simulink model "TxSteering_RxMVDR_4x4_HDL_IQ"  (R2020a)
settings: Solver=FixedStepDiscrete  StartTime=0.0  StopTime=stoptime*0 + inf  RelTol=1e-3
PreLoadFcn:
  | load('iq_bus_obj.mat');
  | model_init
InitFcn:
  | model_init
model workspace (MAT data in the model file):
  socvcb : containers.Map (value not decoded)
values from neighbouring files (symbols this model uses):
  BackSubstitutePrototype = fi(0, matrixdivbacksub_dt)    [model_init.m]
  DataSampleRate = ConverterSampleRate/DecimInterpFactor    (= 245760000)    [model_init.m]
  fc = ConverterSampleRate/4    (= 491520000)    [model_init.m]
  FPGAClkRate = DataSampleRate/VectorSamplingFactor    (= 245760000)    [model_init.m]
  matrixDivDelay = NumberOfCORDICIterations*10 + 86    [model_init.m]
  movavg_bitshift = nextpow2(sqrt(windowSize))    [model_init.m]
  mvdrPipelineDelay = covMatDelay+movAvgDelay+matrixDivDelay+normResponseDelay    [model_init.m]
  NCO_bits = 14    [model_init.m]
  numArrayElements = 4    [model_init.m]
  NumberOfCORDICIterations = matrixdivin_dt.WordLength - 1    [model_init.m]
  S2MM_frame_size = FrameSize*4    (= 40000)    [host_io_init.m]    (also in model_init.m = 1000)
  windowSize = 1024    [model_init.m]
undefined symbols (not defined in the file or in its folder): Fo, Fs, N, physconst
libraries: hdlsllib x268, simulink x53, dspsolvers x1, embreciprocals x1, dsphdlsigops x1
(part 2 of 12)

== system TxSteering_RxMVDR_4x4_HDL_IQ/DUT/Tx Signal Generation/ConcatADCChannels ==
  "Tile1_Ch1_I_Data " : Inport
  Tile1_Ch1_Q_Data : Inport  Port=2
  Tile1_Ch2_I_Data : Inport  Port=3
  Tile1_Ch2_Q_Data : Inport  Port=4
  Tile2_Ch1_I_Data : Inport  Port=5
  Tile2_Ch1_Q_Data : Inport  Port=6
  Tile2_Ch2_I_Data : Inport  Port=7
  Tile2_Ch2_Q_Data : Inport  Port=8
  Valid : Inport  Port=9
  Data Type Conversion : DataTypeConversion  OutDataTypeStr=input_dt  ConvertRealWorld=Stored Integer (SI)
  Real-Imag to Complex{,1..3} (4 alike) : RealImagToComplex
  To Data Bus : Subsystem  mask(To Data Bus){dummy=0}
      mask help: Create a streaming Data Bus from Data and Valid signals.
      mask Display:
      | port_label('input',1,'data');
      | port_label('input',2,'valid');
  Vector Concatenate : Concatenate  NumInputs=4  Mode=Multidimensional array  ConcatenateDimension=2
  DataBusOut : Outport  VectorParamsAs1DForOutWhenUnconnected=off
  wires:
  Real-Imag to Complex/1 -> Vector Concatenate/1
  Real-Imag to Complex1/1 -> Vector Concatenate/2
  Real-Imag to Complex2/1 -> Vector Concatenate/3
  Real-Imag to Complex3/1 -> Vector Concatenate/4
  Vector Concatenate/1 -> Data Type Conversion/1
  Valid/1 -> To Data Bus/2(valid)
  Data Type Conversion/1 -> To Data Bus/1(data)
  To Data Bus/1(bus) -> DataBusOut/1
  "Tile1_Ch1_I_Data "/1 -> Real-Imag to Complex/1
  Tile1_Ch1_Q_Data/1 -> Real-Imag to Complex/2
  Tile1_Ch2_I_Data/1 -> Real-Imag to Complex1/1
  Tile1_Ch2_Q_Data/1 -> Real-Imag to Complex1/2
  Tile2_Ch1_I_Data/1 -> Real-Imag to Complex2/1
  Tile2_Ch1_Q_Data/1 -> Real-Imag to Complex2/2
  Tile2_Ch2_I_Data/1 -> Real-Imag to Complex3/1
  Tile2_Ch2_Q_Data/1 -> Real-Imag to Complex3/2

== system TxSteering_RxMVDR_4x4_HDL_IQ/DUT/Tx Signal Generation/Generate Steering Channels ==
  increment : Inport  Partition=on  PartitionDimension=1  PartitionWidth=1  PartitionOffset=0
  gain : Inport  Port=2  Partition=on  PartitionDimension=1  PartitionWidth=1  PartitionOffset=0
  steeringCoeffs : Inport  Port=3  Partition=on  PartitionDimension=1  PartitionWidth=4  PartitionOffset=0
  Apply Steering Coefficients : Subsystem  TreatAsAtomicUnit=on
  Data Type Conversion : DataTypeConversion  OutDataTypeStr=fixdt(1,16,0)
  For Each : ForEach  DisableCoverage=on
  NCO : Subsystem
  Selector : Selector  InputPortWidth=4  IndexOptions=Index vector (dialog)  Indices=1  OutputSizes=1
  dataOut : Outport  ConcatenationDimension=1
  validOut : Outport  Port=2  ConcatenationDimension=1
  wires:
  Data Type Conversion/1 -> dataOut/1
  Selector/1 -> validOut/1
  steeringCoeffs/1 -> Apply Steering Coefficients/3(coeffIn)
  increment/1 -> NCO/1(increment)
  Apply Steering Coefficients/1(dataOut) -> Data Type Conversion/1
  Apply Steering Coefficients/2(validOut) -> Selector/1
  NCO/1(dataOut) -> Apply Steering Coefficients/1(dataIn)
  gain/1 -> NCO/2(gain)
  NCO/2(validOut) -> Apply Steering Coefficients/2(validIn)

== system TxSteering_RxMVDR_4x4_HDL_IQ/AXI4Stream_DMA_S2MM/ForCalibration/Unpack Complex/For Each Subsystem ==
  In1 : Inport  Partition=on  PartitionDimension=1  PartitionWidth=1  PartitionOffset=0
  For Each : ForEach  DisableCoverage=on
  Out1 : Outport  ConcatenationDimension=1
  wires:
  In1/1 -> Out1/1

== system TxSteering_RxMVDR_4x4_HDL_IQ/AXI4Stream_DMA_S2MM/ForCalibration/Unpack Complex/Subsystem ==
  In1 : Inport
  Bit Slice : hdlsllib/Logic and Bit Operations/Bit Slice  lidx=15  ridx=0
      settings: SourceProductBaseCode=SL
  Bit Slice1 : hdlsllib/Logic and Bit Operations/Bit Slice  lidx=31  ridx=16
      settings: SourceProductBaseCode=SL
  Bit Slice2 : hdlsllib/Logic and Bit Operations/Bit Slice  lidx=47  ridx=32
      settings: SourceProductBaseCode=SL
  Bit Slice3 : hdlsllib/Logic and Bit Operations/Bit Slice  lidx=63  ridx=48
      settings: SourceProductBaseCode=SL
  Data Type Conversion{1..4} (4 alike) : DataTypeConversion  OutDataTypeStr=fixdt(1,16,15)  ConvertRealWorld=Stored Integer (SI)
  Out1 : Outport
  Out2 : Outport  Port=2
  Out3 : Outport  Port=3
  Out4 : Outport  Port=4
  wires:
  Bit Slice1/1 -> Data Type Conversion1/1
  In1/1 -> Bit Slice/1, Bit Slice1/1, Bit Slice3/1, Bit Slice2/1
  Bit Slice2/1 -> Data Type Conversion3/1
  Bit Slice/1 -> Data Type Conversion2/1
  Bit Slice3/1 -> Data Type Conversion4/1
  Data Type Conversion2/1 -> Out1/1
  Data Type Conversion1/1 -> Out2/1
  Data Type Conversion3/1 -> Out3/1
  Data Type Conversion4/1 -> Out4/1

== system TxSteering_RxMVDR_4x4_HDL_IQ/AXI4Stream_DMA_S2MM/ForCalibration/Unpack Complex/Subsystem1 ==
  In1 : Inport
  Bit Slice : hdlsllib/Logic and Bit Operations/Bit Slice  lidx=15  ridx=0
      settings: SourceProductBaseCode=SL
  Bit Slice1 : hdlsllib/Logic and Bit Operations/Bit Slice  lidx=31  ridx=16
      settings: SourceProductBaseCode=SL
  Bit Slice2 : hdlsllib/Logic and Bit Operations/Bit Slice  lidx=47  ridx=32
      settings: SourceProductBaseCode=SL
  Bit Slice3 : hdlsllib/Logic and Bit Operations/Bit Slice  lidx=63  ridx=48
      settings: SourceProductBaseCode=SL
  Data Type Conversion{1..4} (4 alike) : DataTypeConversion  OutDataTypeStr=fixdt(1,16,15)  ConvertRealWorld=Stored Integer (SI)
  Out1 : Outport
  Out2 : Outport  Port=2
  Out3 : Outport  Port=3
  Out4 : Outport  Port=4
  wires:
  Bit Slice3/1 -> Data Type Conversion1/1
  Bit Slice2/1 -> Data Type Conversion2/1
  Bit Slice/1 -> Data Type Conversion3/1
  In1/1 -> Bit Slice2/1, Bit Slice3/1, Bit Slice1/1, Bit Slice/1
  Bit Slice1/1 -> Data Type Conversion4/1
  Data Type Conversion2/1 -> Out3/1
  Data Type Conversion1/1 -> Out4/1
  Data Type Conversion3/1 -> Out1/1
  Data Type Conversion4/1 -> Out2/1

== system TxSteering_RxMVDR_4x4_HDL_IQ/DUT/ConcatADCChannels/Apply Calibration Coefficients/For Each Subsystem ==
  dataIn : Inport  Partition=on  PartitionDimension=1  PartitionWidth=1  PartitionOffset=0
  validIn : Inport  Port=2
  coeffIn : Inport  Port=3  Partition=on  PartitionDimension=1  PartitionWidth=1  PartitionOffset=0
  For Each : ForEach  DisableCoverage=on
  HDL Complex Multiplier : Subsystem
  dataOut : Outport  ConcatenationDimension=1
  validOut : Outport  Port=2  ConcatenationDimension=1
  wires:
  dataIn/1 -> HDL Complex Multiplier/1(z1)
  coeffIn/1 -> HDL Complex Multiplier/2(z2)
  validIn/1 -> HDL Complex Multiplier/3(validIn)
  HDL Complex Multiplier/1(z) -> dataOut/1
  HDL Complex Multiplier/2(validOut) -> validOut/1

== system TxSteering_RxMVDR_4x4_HDL_IQ/DUT/MVDR/Compute Weight Vector/Matrix Left Divide ==
  A : Inport
  B : Inport  Port=2
  validIn : Inport  Port=3
  CORDIC : Subsystem  VariantControl=HDL
  QR Solver : Subsystem  VariantControl=Simulation
  x : Outport
  validOut : Outport  Port=2
  ready : Outport  Port=3

== system TxSteering_RxMVDR_4x4_HDL_IQ/DUT/MVDR/Form Beam/Parallel Complex Multiply ==
  z1 : Inport  Partition=on  PartitionDimension=1  PartitionWidth=1  PartitionOffset=0
  z2 : Inport  Port=2  Partition=on  PartitionDimension=1  PartitionWidth=1  PartitionOffset=0
  For Each : ForEach  DisableCoverage=on
  HDL Complex Multiply : Subsystem  mask(HDL Complex Multiplier (3 Multiply, 5 Add)){D1=2, D2=1, D3=1, D4=1, D5=1}
      mask help:
      | Xilinx devices:
      | - Set D1 = 1 or 2 to trade off speed & FF resources
      | - Set D2-D5 = 1 to fully leverage DSP48 pipelines
      | - Use sync reset
      |
      | Intel FPGAs:
      | - Set D1 = 1 or 2 depending on device family
      | - Set D5 = 1; D2, D3, D4 = 0
      | - Use async reset
      mask init:
      | delay = D1+D2+D3+D4+D5;
      mask Display:
      | fprintf('Delay=%d',delay);
      | port_label('input',1,'z1');
      | port_label('input',2,'z2');
  z : Outport  ConcatenationDimension=1
  wires:
  z1/1 -> HDL Complex Multiply/1(In1)
  z2/1 -> HDL Complex Multiply/2(In2)
  HDL Complex Multiply/1(Out1) -> z/1

== system TxSteering_RxMVDR_4x4_HDL_IQ/DUT/MVDR/Form Beam/Tree Sum ==
  In1 : Inport
  Add : Sum
  Add1 : Sum
  Add2 : Sum
  Delay : Delay  DelayLength=1
  Delay1 : Delay  DelayLength=1
  Delay2 : Delay  DelayLength=1
  Demux : Demux
  Out1 : Outport
  wires:
  Add/1 -> Delay2/1
  Add1/1 -> Delay1/1
  In1/1 -> Demux/1
  Demux/1 -> Add/1
  Demux/2 -> Add/2
  Demux/3 -> Add1/1
  Demux/4 -> Add1/2
  Add2/1 -> Delay/1
  Delay/1 -> Out1/1
  Delay1/1 -> Add2/2
  Delay2/1 -> Add2/1

== system TxSteering_RxMVDR_4x4_HDL_IQ/DUT/MVDR/Form Covariance Matrix/Matrix Multiply Partitioned ==
  x : Inport
  x_conj : Inport  Port=2
  Partition x_conj : Subsystem
  C : Outport
  wires:
  x/1 -> Partition x_conj/1(x)
  x_conj/1 -> Partition x_conj/2(x_conj)
  Partition x_conj/1(C) -> C/1

== system TxSteering_RxMVDR_4x4_HDL_IQ/DUT/MVDR/Moving Average/Wait for Running Sum Init ==
  In1 : Inport
  Compare To Constant : simulink/Logic and Bit Operations/Compare To Constant  relop=<  const=windowSize  OutDataTypeStr=boolean
  HDL Counter : hdlsllib/Sources/HDL Counter  CountType=Free running  CountInit=0  CountStep=1  CountMax=25  CountFromType=Initial value  CountFrom=0  CountResetPort=off  CountLoadPort=off  CountEnbPort=on  CountDirPort=off  CountDataType=Unsigned  CountWordLen=nextpow2(windowSize)+1  CountFracLen=0  CountSampTime=1
  Logical Operator : Logic  IconShape=distinctive  AllPortsSameDT=off  OutDataTypeStr=boolean
  Logical Operator1 : Logic  IconShape=distinctive  AllPortsSameDT=off  OutDataTypeStr=boolean
  Logical Operator2 : Logic  Operator=NOT  IconShape=distinctive  AllPortsSameDT=off  OutDataTypeStr=boolean
  Out1 : Outport
  wires:
  Logical Operator2/1 -> Logical Operator/2
  Logical Operator1/1 -> HDL Counter/1
  Compare To Constant/1 -> Logical Operator1/2, Logical Operator2/1
  Logical Operator/1 -> Out1/1
  HDL Counter/1 -> Compare To Constant/1
  In1/1 -> Logical Operator1/1, Logical Operator/1

== system TxSteering_RxMVDR_4x4_HDL_IQ/DUT/MVDR/Normalize Response/MVDR Weight Update ==
  Steering Vector : Inport
  x : Inport  Port=2
  validIn : Inport  Port=3
  Delay{,1,3..6} (6 alike) : Delay  DelayLength=1
  Delay2 : Delay  DelayLength=8
  Inner Product : Subsystem
  Vector / Scalar Divide : Subsystem
  w : Outport
  validOut : Outport  Port=2
  wires:
  x/1 -> Delay3/1
  Vector / Scalar Divide/1(w) -> w/1
  Delay4/1 -> Inner Product/1(u)
  Inner Product/1(y) -> Delay5/1
  Delay6/1 -> Vector / Scalar Divide/1(x)
  Delay/1 -> Vector / Scalar Divide/3(validIn)
  Steering Vector/1 -> Delay4/1
  Delay3/1 -> Delay2/1, Inner Product/2(v)
  Delay5/1 -> Vector / Scalar Divide/2(y)
  Inner Product/2(validOut) -> Delay/1
  validIn/1 -> Delay1/1
  Vector / Scalar Divide/2(validOut) -> validOut/1
  Delay1/1 -> Inner Product/3(validIn)
  Delay2/1 -> Delay6/1

== system TxSteering_RxMVDR_4x4_HDL_IQ/DUT/MVDR/Subsystem/RepackageInput ==
  In1 : Inport
  Bitconcat : Subsystem
  Bus Creator : BusCreator  Inputs=2
  Bus Selector : BusSelector  OutputSignals=data,valid
  Out1 : Outport
  wires:
  In1/1 -> Bus Selector/1
  Bus Creator/1 -> Out1/1
  Bus Selector/2 -> Bus Creator/2  "<valid>"
  Bus Selector/1 -> Bitconcat/1(<data>)  "<data>"
  Bitconcat/1(Out1) -> Bus Creator/1  "data"

== system TxSteering_RxMVDR_4x4_HDL_IQ/DUT/MVDR/Subsystem/RepackageMVDR ==
  In3 : Inport
  Bit Concat : hdlsllib/Logic and Bit Operations/Bit Concat  numInputs=2
  Bus Creator : BusCreator  Inputs=2
  Bus Selector : BusSelector  OutputSignals=data,valid
  Complex to Real-Imag : ComplexToRealImag
  Data Type Conversion1 : DataTypeConversion  OutDataTypeStr=fixdt(0,128,0)  ConvertRealWorld=Stored Integer (SI)
  Out1 : Outport
  wires:
  Bit Concat/1 -> Data Type Conversion1/1
  Data Type Conversion1/1 -> Bus Creator/1  "data"
  Bus Selector/1 -> Complex to Real-Imag/1  "<data>"
  Complex to Real-Imag/2 -> Bit Concat/1
  Bus Selector/2 -> Bus Creator/2  "<valid>"
  In3/1 -> Bus Selector/1
  Bus Creator/1 -> Out1/1
  Complex to Real-Imag/1 -> Bit Concat/2

== system TxSteering_RxMVDR_4x4_HDL_IQ/DUT/Rx Data Capture/AXI4-Lite Initial Value/Set_Latch ==
  S : Inport
  Logical Operator5 : Logic  Operator=OR  IconShape=distinctive  AllPortsSameDT=off  OutDataTypeStr=boolean
  Unit Delay : UnitDelay  SampleTime=-1  HasFrameUpgradeWarning=on
  Q : Outport  VectorParamsAs1DForOutWhenUnconnected=off
  wires:
  Logical Operator5/1 -> Unit Delay/1
  S/1 -> Logical Operator5/1
  Unit Delay/1 -> Q/1, Logical Operator5/2

== system TxSteering_RxMVDR_4x4_HDL_IQ/DUT/Rx Data Capture/EnableConsecutiveFrames/sr_latch ==
  S : Inport
  R : Inport  Port=2
  Logical Operator1 : Logic  IconShape=distinctive  AllPortsSameDT=off  OutDataTypeStr=boolean
  Logical Operator2 : Logic  Operator=NOT  IconShape=distinctive  AllPortsSameDT=off  OutDataTypeStr=boolean
  Logical Operator9 : Logic  Operator=OR  IconShape=distinctive  AllPortsSameDT=off  OutDataTypeStr=boolean
  Unit Delay1 : UnitDelay  SampleTime=-1  HasFrameUpgradeWarning=on
  Q : Outport  VectorParamsAs1DForOutWhenUnconnected=off
  wires:
  S/1 -> Logical Operator9/1
  R/1 -> Logical Operator2/1
  Logical Operator2/1 -> Logical Operator1/1
  Unit Delay1/1 -> Logical Operator1/2, Q/1
  Logical Operator9/1 -> Unit Delay1/1
  Logical Operator1/1 -> Logical Operator9/2

== system TxSteering_RxMVDR_4x4_HDL_IQ/DUT/Rx Data Capture/Stream FIFO /hdl_fwft_fifo ==
  data_i : Inport
  push : Inport  Port=2
  rd_ack : Inport  Port=3
  Compare To Constant : simulink/Logic and Bit Operations/Compare To Constant  relop=>=  const=FIFO_DEPTH-AFULL_THRESH  OutDataTypeStr=boolean
  HDL FIFO : hdlsllib/HDL RAMs/HDL FIFO  fifo_size=FIFO_DEPTH  mode=FWFT  ratio=1  push_msg=Error  pop_msg=Ignore  show_empty=on  show_full=on  show_num=on  LabelModeActiveChoice_Mode=FWFT
      settings: SourceProductBaseCode=SL
  Logical Operator1 : Logic  Operator=NOT  IconShape=distinctive  AllPortsSameDT=off  OutDataTypeStr=boolean
  Logical Operator2 : Logic  IconShape=distinctive  AllPortsSameDT=off  OutDataTypeStr=boolean
  data_o : Outport  VectorParamsAs1DForOutWhenUnconnected=off
  empty : Outport  Port=2  VectorParamsAs1DForOutWhenUnconnected=off
  num : Outport  Port=3  VectorParamsAs1DForOutWhenUnconnected=off
  full : Outport  Port=4  VectorParamsAs1DForOutWhenUnconnected=off
  afull : Outport  Port=5  VectorParamsAs1DForOutWhenUnconnected=off
  wires:
  Compare To Constant/1 -> afull/1
  data_i/1 -> HDL FIFO/1
  push/1 -> Logical Operator2/1
  Logical Operator2/1 -> HDL FIFO/2
  Logical Operator1/1 -> Logical Operator2/2
  HDL FIFO/3 -> Logical Operator1/1, full/1
  HDL FIFO/4 -> Compare To Constant/1, num/1
  HDL FIFO/2 -> empty/1
  HDL FIFO/1 -> data_o/1
  rd_ack/1 -> HDL FIFO/3

== system TxSteering_RxMVDR_4x4_HDL_IQ/DUT/Tx Signal Generation/ConcatADCChannels/To Data Bus ==
  data : Inport
  valid : Inport  Port=2
  Bus Creator : BusCreator  Inputs=2
  bus : Outport  VectorParamsAs1DForOutWhenUnconnected=off
  wires:
  Bus Creator/1 -> bus/1
  data/1 -> Bus Creator/1  "data"
  valid/1 -> Bus Creator/2  "valid"

== system TxSteering_RxMVDR_4x4_HDL_IQ/DUT/Tx Signal Generation/Generate Steering Channels/Apply Steering Coefficients ==
  dataIn : Inport
  validIn : Inport  Port=2
  coeffIn : Inport  Port=3  Partition=on  PartitionDimension=1  PartitionWidth=1  PartitionOffset=0
  For Each : ForEach  DisableCoverage=on
  HDL Complex Multiplier : Subsystem
  dataOut : Outport  ConcatenationDimension=1
  validOut : Outport  Port=2  ConcatenationDimension=1
  wires:
  dataIn/1 -> HDL Complex Multiplier/1(z1)
  coeffIn/1 -> HDL Complex Multiplier/2(z2)
  validIn/1 -> HDL Complex Multiplier/3(validIn)
  HDL Complex Multiplier/1(z) -> dataOut/1
  HDL Complex Multiplier/2(validOut) -> validOut/1

== system TxSteering_RxMVDR_4x4_HDL_IQ/DUT/Tx Signal Generation/Generate Steering Channels/NCO ==
  increment : Inport
  gain : Inport  Port=2
  Constant : Constant  Value=true  SampleTime=-1
  Data Type Duplicate : DataTypeDuplicate
  Data Type Conversion : DataTypeConversion  OutDataTypeStr=fixdt(1,16,14)
  Data Type Conversion1 : DataTypeConversion
  Data Type Conversion2 : DataTypeConversion  OutDataTypeStr=int16  ConvertRealWorld=Stored Integer (SI)  LockScale=on
  NCO HDL Optimized : dsphdlsigops/NCO HDL Optimized  PhaseIncrementSource=Input port  PhaseIncrement=round(Fo*(2^N)/Fs)  PhaseOffsetSource=Property  PhaseOffset=0  DitherSource=Property  NumDitherBits=4  SamplesPerFrame=1  LUTCompress=on  ResetAction=off  Waveform=Complex exponential  PhasePort=off  SimulateUsing=Code generation  AccumulatorWL=NCO_bits  PhaseQuantization=off  NumQuantizerAccumulatorBits=12  OutputDataType=Binary point scaling  OutputWL=NCO_bits  OutputFL=NCO_bits-2
      settings: SourceProductBaseCode=DS
  PipelineDelay : Delay
  PipelineDelay1 : Delay
  PipelineDelay2 : Delay  DelayLength=1
  PipelineDelay3 : Delay
  PipelineDelay4 : Delay  DelayLength=1
  Product : Product
  dataOut : Outport
  validOut : Outport  Port=2  VectorParamsAs1DForOutWhenUnconnected=off
  wires:
  NCO HDL Optimized/1 -> Data Type Conversion/1
  NCO HDL Optimized/2 -> PipelineDelay3/1
  increment/1 -> NCO HDL Optimized/1
  Data Type Conversion/1 -> Data Type Conversion2/1
  gain/1 -> PipelineDelay/1
  PipelineDelay/1 -> Product/1
  PipelineDelay1/1 -> Product/2
  Product/1 -> PipelineDelay2/1
  PipelineDelay2/1 -> Data Type Conversion1/1
  Data Type Conversion1/1 -> dataOut/1, Data Type Duplicate/2
  PipelineDelay3/1 -> PipelineDelay4/1
  PipelineDelay4/1 -> validOut/1
  Constant/1 -> NCO HDL Optimized/2
  Data Type Conversion2/1 -> Data Type Duplicate/1, PipelineDelay1/1

== system TxSteering_RxMVDR_4x4_HDL_IQ/DUT/ConcatADCChannels/Apply Calibration Coefficients/For Each Subsystem/HDL Complex Multiplier ==
  z1 : Inport
  z2 : Inport  Port=2
  validIn : Inport  Port=3
  Add1 : Sum  Inputs=+-
  Add2 : Sum
  Complex to Real-Imag1 : ComplexToRealImag
  Complex to Real-Imag2 : ComplexToRealImag
  Delay{1,4,7..9,11} (6 alike) : Delay  DelayLength=1  InitialCondition=0  InputProcessing=Columns as channels (frame based)
  Delay{2..3,5..6,10} (5 alike) : Delay  InitialCondition=0  InputProcessing=Columns as channels (frame based)
  Product{,1,3..4} (4 alike) : Product
  Real-Imag to Complex : RealImagToComplex
  z : Outport  VectorParamsAs1DForOutWhenUnconnected=off
  validOut : Outport  Port=2  VectorParamsAs1DForOutWhenUnconnected=off
  wires:
  Add2/1 -> Delay4/1
  Add1/1 -> Delay1/1
  Complex to Real-Imag2/2 -> Product1/2, Product3/2
  Complex to Real-Imag1/2 -> Product1/1, Product4/2
  Complex to Real-Imag2/1 -> Product/2, Product4/1
  Complex to Real-Imag1/1 -> Product/1, Product3/1
  Product/1 -> Delay2/1
  Product1/1 -> Delay3/1
  Product3/1 -> Delay5/1
  Product4/1 -> Delay6/1
  Delay2/1 -> Add1/1
  Delay3/1 -> Add1/2
  Delay6/1 -> Add2/2
  Real-Imag to Complex/1 -> z/1
  z1/1 -> Delay7/1
  z2/1 -> Delay8/1
  Delay5/1 -> Add2/1
  Delay1/1 -> Real-Imag to Complex/1
  Delay4/1 -> Real-Imag to Complex/2
  Delay7/1 -> Complex to Real-Imag1/1
  Delay8/1 -> Complex to Real-Imag2/1
  validIn/1 -> Delay9/1
  Delay9/1 -> Delay10/1
  Delay10/1 -> Delay11/1
  Delay11/1 -> validOut/1

== system TxSteering_RxMVDR_4x4_HDL_IQ/DUT/MVDR/Compute Weight Vector/Matrix Left Divide/CORDIC ==
  A : Inport
  B : Inport  Port=2
  validIn : Inport  Port=3
  4x4 Complex CORDIC Matrix Left Divide : Subsystem  TreatAsAtomicUnit=on  mask(4x4 Complex CORDIC Matrix Left Divide){NumberOfCORDICIterations=NumberOfCORDICIterations, OutputPrototype=BackSubstitutePrototype}
      mask prompts: NumberOfCORDICIterations "Number of CORDIC Iterations"; OutputPrototype "Back-Substitute Prototype"
      mask help: Solve AX=B using QR factorization using CORDIC. Matrix A must be 4x4. Matrix B must have 4 rows.
  Demux : Demux
  Reshape : Reshape  OutputDimensionality=Customize  OutputDimensions=[4,4]
  Selector : Selector  NumberOfDimensions=2  InputPortWidth=3  IndexOptions=Index vector (dialog),Select all  Indices=1,1  OutputSizes=1,1
  Selector1 : Selector  NumberOfDimensions=2  InputPortWidth=3  IndexOptions=Index vector (dialog),Select all  Indices=2,1  OutputSizes=1,1
  Selector2 : Selector  NumberOfDimensions=2  InputPortWidth=3  IndexOptions=Index vector (dialog),Select all  Indices=3,1  OutputSizes=1,1
  Selector3 : Selector  NumberOfDimensions=2  InputPortWidth=3  IndexOptions=Index vector (dialog),Select all  Indices=4,1  OutputSizes=1,1
  Vector Concatenate : Concatenate  NumInputs=4  Mode=Multidimensional array
  x : Outport
  validOut : Outport  Port=2
  ready : Outport  Port=3
  wires:
  Selector/1 -> 4x4 Complex CORDIC Matrix Left Divide/1(a1)
  4x4 Complex CORDIC Matrix Left Divide/2(x2) -> Vector Concatenate/2
  4x4 Complex CORDIC Matrix Left Divide/1(x1) -> Vector Concatenate/1
  4x4 Complex CORDIC Matrix Left Divide/3(x3) -> Vector Concatenate/3
  4x4 Complex CORDIC Matrix Left Divide/4(x4) -> Vector Concatenate/4
  4x4 Complex CORDIC Matrix Left Divide/6(ready) -> ready/1
  Selector1/1 -> 4x4 Complex CORDIC Matrix Left Divide/2(a2)
  Selector2/1 -> 4x4 Complex CORDIC Matrix Left Divide/3(a3)
  Selector3/1 -> 4x4 Complex CORDIC Matrix Left Divide/4(a4)
  Demux/1 -> 4x4 Complex CORDIC Matrix Left Divide/5(b1)
  Demux/4 -> 4x4 Complex CORDIC Matrix Left Divide/8(b4)
  Demux/2 -> 4x4 Complex CORDIC Matrix Left Divide/6(b2)
  Demux/3 -> 4x4 Complex CORDIC Matrix Left Divide/7(b3)
  4x4 Complex CORDIC Matrix Left Divide/5(validOut) -> validOut/1
  Reshape/1 -> Selector1/1, Selector2/1, Selector3/1, Selector/1
  A/1 -> Reshape/1
  B/1 -> Demux/1
  validIn/1 -> 4x4 Complex CORDIC Matrix Left Divide/9(validIn)
  Vector Concatenate/1 -> x/1

== system TxSteering_RxMVDR_4x4_HDL_IQ/DUT/MVDR/Compute Weight Vector/Matrix Left Divide/QR Solver ==
  A : Inport
  B : Inport  Port=2
  validIn : Inport  Port=3
  Data Type Conversion : DataTypeConversion  OutDataTypeStr=single
  Data Type Conversion1 : DataTypeConversion  OutDataTypeStr=single
  Data Type Conversion2 : DataTypeConversion  OutDataTypeStr=matrixdivbacksub_dt
  Delay1 : Delay  DelayLength=matrixDivDelay
  Delay6 : Delay  DelayLength=matrixDivDelay
  Emulate CORDIC Ready : Subsystem
  Reshape : Reshape  OutputDimensionality=Customize  OutputDimensions=[4,4]
  Reshape1 : Reshape  OutputDimensionality=Customize  OutputDimensions=[4,1]
  Subsystem : Subsystem
  x : Outport
  validOut : Outport  Port=2
  ready : Outport  Port=3
  wires:
  B/1 -> Reshape1/1
  A/1 -> Reshape/1
  validIn/1 -> Emulate CORDIC Ready/1(In1), Subsystem/Enable, Delay1/1
  Reshape/1 -> Data Type Conversion/1
  Emulate CORDIC Ready/1(Out1) -> ready/1
  Delay6/1 -> Data Type Conversion2/1
  Delay1/1 -> validOut/1
  Data Type Conversion/1 -> Subsystem/1(In1)
  Data Type Conversion1/1 -> Subsystem/2(In2)
  Subsystem/1(Out1) -> Delay6/1
  Reshape1/1 -> Data Type Conversion1/1
  Data Type Conversion2/1 -> x/1

== system TxSteering_RxMVDR_4x4_HDL_IQ/DUT/MVDR/Form Beam/Parallel Complex Multiply/HDL Complex Multiply ==
  note: Xilinx devices:
      | - Set D1 = 1 or 2 to trade off speed & FF resources
      | - Set D2-D5 = 1 to fully leverage DSP48 pipelines
      | - Use sync reset
      |
      | Intel FPGAs:
      | - Set D1 = 1 or 2 depending on device family
      | - Set D5 = 1; D2, D3, D4 = 0
      | - Use async reset
  In1 : Inport
  In2 : Inport  Port=2
  Add1 : Sum
  Add2 : Sum  Inputs=+-
  Add3 : Sum
  Add4 : Sum  Inputs=-+
  Add5 : Sum
  Complex to Real-Imag : ComplexToRealImag
  Complex to Real-Imag1 : ComplexToRealImag
  D1_1 : Delay  DelayLength=D1
  D1_2 : Delay  DelayLength=D1
  D2_{1..6} (6 alike) : Delay  DelayLength=D2
  D3_{1..5} (5 alike) : Delay  DelayLength=D3
  D4_1 : Delay  DelayLength=D4
  D4_2 : Delay  DelayLength=D4
  D4_3 : Delay  DelayLength=D4
  D5_1 : Delay  DelayLength=D5
  D5_2 : Delay  DelayLength=D5
  Product1 : Product
  Product2 : Product
  Product3 : Product
  Real-Imag to Complex : RealImagToComplex
  Out1 : Outport  VectorParamsAs1DForOutWhenUnconnected=off
  wires:
  Real-Imag to Complex/1 -> Out1/1
  In2/1 -> D1_2/1
  Complex to Real-Imag1/1 -> Add3/1, D2_4/1  "C"
  Complex to Real-Imag1/2 -> Add3/2, D2_3/1  "D"
  Product1/1 -> D4_1/1  "X"
  Product2/1 -> D4_2/1  "Y"
  Product3/1 -> D3_5/1  "Z"
  Add4/1 -> D5_1/1
  Add5/1 -> D5_2/1
  D5_1/1 -> Real-Imag to Complex/1
  D5_2/1 -> Real-Imag to Complex/2
  D4_1/1 -> Add4/1
  D4_2/1 -> Add5/1
  D3_5/1 -> D4_3/1
  Add1/1 -> D3_1/1
  Add3/1 -> D2_6/1
  Add2/1 -> D3_3/1
  Complex to Real-Imag/1 -> D2_5/1, D2_1/1  "A"
  Complex to Real-Imag/2 -> D2_2/1  "B"
  D3_1/1 -> Product1/1
  D2_6/1 -> Product3/2
  D3_3/1 -> Product2/1
  D4_3/1 -> Add4/2, Add5/2
  D3_4/1 -> Product2/2
  D3_2/1 -> Product1/2
  D2_4/1 -> D3_4/1
  D2_3/1 -> D3_2/1
  D2_5/1 -> Product3/1
  D2_2/1 -> Add1/2, Add2/1
  D2_1/1 -> Add2/2, Add1/1
  In1/1 -> D1_1/1
  D1_1/1 -> Complex to Real-Imag/1
  D1_2/1 -> Complex to Real-Imag1/1

== system TxSteering_RxMVDR_4x4_HDL_IQ/DUT/MVDR/Form Covariance Matrix/Matrix Multiply Partitioned/Partition x_conj ==
  x : Inport
  x_conj : Inport  Port=2  Partition=on  PartitionDimension=1  PartitionWidth=1  PartitionOffset=0
  For Each : ForEach  DisableCoverage=on
  Partition x : Subsystem  TreatAsAtomicUnit=on
  C : Outport  ConcatenationDimension=1
  wires:
  x_conj/1 -> Partition x/2(x_conj_elem)
  x/1 -> Partition x/1(x)
  Partition x/1(C_col) -> C/1

== system TxSteering_RxMVDR_4x4_HDL_IQ/DUT/MVDR/Normalize Response/MVDR Weight Update/Inner Product ==
  u : Inport
  v : Inport  Port=2
  validIn : Inport  Port=3
  Conjugate : Math  Operator=conj  SignedPower=on  RndMeth=Zero  SaturateOnIntegerOverflow=on
  Delay : Delay  DelayLength=1
  Delay1 : Delay  DelayLength=6
  Delay2 : Delay  DelayLength=ceil(log2(numArrayElements))
  Delay4 : Delay  DelayLength=1
  Element-wise complex product : Subsystem  TreatAsAtomicUnit=on
  Tree Sum with Distributed Pipelining : Subsystem
  y : Outport
  validOut : Outport  Port=2
  wires:
  v/1 -> Conjugate/1
  u/1 -> Element-wise complex product/2(v)
  validIn/1 -> Delay1/1
  Element-wise complex product/1(y) -> Delay/1
  Delay2/1 -> validOut/1
  Delay1/1 -> Delay4/1
  Delay4/1 -> Delay2/1
  Conjugate/1 -> Element-wise complex product/1(u)
  Delay/1 -> Tree Sum with Distributed Pipelining/1(In1)
  Tree Sum with Distributed Pipelining/1(Out1) -> y/1

== system TxSteering_RxMVDR_4x4_HDL_IQ/DUT/MVDR/Normalize Response/MVDR Weight Update/Vector // Scalar Divide ==
  x : Inport
  y : Inport  Port=2
  validIn : Inport  Port=3
  Complex to Real-Imag : ComplexToRealImag  Output=Real
  Data Type Conversion : DataTypeConversion  OutDataTypeStr=fixdt(1,18,16)
  Delay{1..6,11..13} (9 alike) : Delay  DelayLength=1
  Delay{7..10} (4 alike) : Delay
  Delay14 : Delay  DelayLength=34
  MATLAB Function : MATLAB Function  TreatAsAtomicUnit=on
  Normalized Reciprocal HDL Optimized : embreciprocals/Normalized Reciprocal HDL Optimized
      settings: SourceProductBaseCode=PO
  Product : Product  OutDataTypeStr=Inherit: Same as first input
  w : Outport
  validOut : Outport  Port=2
  wires:
  Delay2/1 -> MATLAB Function/2(e)
  y/1 -> Complex to Real-Imag/1
  Delay12/1 -> Data Type Conversion/1
  Complex to Real-Imag/1 -> Normalized Reciprocal HDL Optimized/1
  Delay13/1 -> Delay7/1
  Normalized Reciprocal HDL Optimized/2 -> Delay11/1
  Normalized Reciprocal HDL Optimized/1 -> Delay12/1
  Delay1/1 -> MATLAB Function/1(y)
  validIn/1 -> Normalized Reciprocal HDL Optimized/2
  Product/1 -> Delay1/1
  Delay11/1 -> Delay9/1
  MATLAB Function/1(w) -> Delay3/1
  Normalized Reciprocal HDL Optimized/3 -> Delay4/1
  Delay3/1 -> w/1
  Delay4/1 -> Delay10/1
  Delay5/1 -> Delay6/1
  Delay6/1 -> validOut/1
  x/1 -> Delay14/1
  Data Type Conversion/1 -> Delay8/1
  Delay7/1 -> Product/1
  Delay8/1 -> Product/2
  Delay9/1 -> Delay2/1
  Delay10/1 -> Delay5/1
  Delay14/1 -> Delay13/1

== system TxSteering_RxMVDR_4x4_HDL_IQ/DUT/MVDR/Subsystem/RepackageInput/Bitconcat ==
  <data> : Inport
  Bit Concat : hdlsllib/Logic and Bit Operations/Bit Concat  numInputs=4
  For Each Subsystem : Subsystem  TreatAsAtomicUnit=on
  Selector : Selector  InputPortWidth=4  IndexOptions=Index vector (dialog)  Indices=1  OutputSizes=1
  Selector1 : Selector  InputPortWidth=4  IndexOptions=Index vector (dialog)  Indices=2  OutputSizes=1
  Selector2 : Selector  InputPortWidth=4  IndexOptions=Index vector (dialog)  Indices=3  OutputSizes=1
  Selector3 : Selector  InputPortWidth=4  IndexOptions=Index vector (dialog)  Indices=4  OutputSizes=1
  Out1 : Outport
  wires:
  Selector3/1 -> Bit Concat/4
  Selector1/1 -> Bit Concat/2
  Selector/1 -> Bit Concat/1
  Selector2/1 -> Bit Concat/3
  <data>/1 -> For Each Subsystem/1(In1)
  Bit Concat/1 -> Out1/1
  For Each Subsystem/1(Out1) -> Selector3/1, Selector2/1, Selector1/1, Selector/1

== system TxSteering_RxMVDR_4x4_HDL_IQ/DUT/Tx Signal Generation/Generate Steering Channels/Apply Steering Coefficients/HDL Complex Multiplier ==
  z1 : Inport
  z2 : Inport  Port=2
  validIn : Inport  Port=3
  Add1 : Sum  Inputs=+-
  Add2 : Sum
  Complex to Real-Imag1 : ComplexToRealImag
  Complex to Real-Imag2 : ComplexToRealImag
  Delay{1,4,7..9,11} (6 alike) : Delay  DelayLength=1  InitialCondition=0  InputProcessing=Columns as channels (frame based)
  Delay{2..3,5..6,10} (5 alike) : Delay  InitialCondition=0  InputProcessing=Columns as channels (frame based)
  Product{,1,3..4} (4 alike) : Product
  Real-Imag to Complex : RealImagToComplex
  z : Outport  VectorParamsAs1DForOutWhenUnconnected=off
  validOut : Outport  Port=2  VectorParamsAs1DForOutWhenUnconnected=off
  wires:
  Add2/1 -> Delay4/1
  Add1/1 -> Delay1/1
  Complex to Real-Imag2/2 -> Product1/2, Product3/2
  Complex to Real-Imag1/2 -> Product1/1, Product4/2
  Complex to Real-Imag2/1 -> Product/2, Product4/1
  Complex to Real-Imag1/1 -> Product/1, Product3/1
  Product/1 -> Delay2/1
  Product1/1 -> Delay3/1
  Product3/1 -> Delay5/1
  Product4/1 -> Delay6/1
  Delay2/1 -> Add1/1
  Delay3/1 -> Add1/2
  Delay6/1 -> Add2/2
  Real-Imag to Complex/1 -> z/1
  z1/1 -> Delay7/1
  z2/1 -> Delay8/1
  Delay5/1 -> Add2/1
  Delay1/1 -> Real-Imag to Complex/1
  Delay4/1 -> Real-Imag to Complex/2
  Delay7/1 -> Complex to Real-Imag1/1
  Delay8/1 -> Complex to Real-Imag2/1
  validIn/1 -> Delay9/1
  Delay9/1 -> Delay10/1
  Delay10/1 -> Delay11/1
  Delay11/1 -> validOut/1

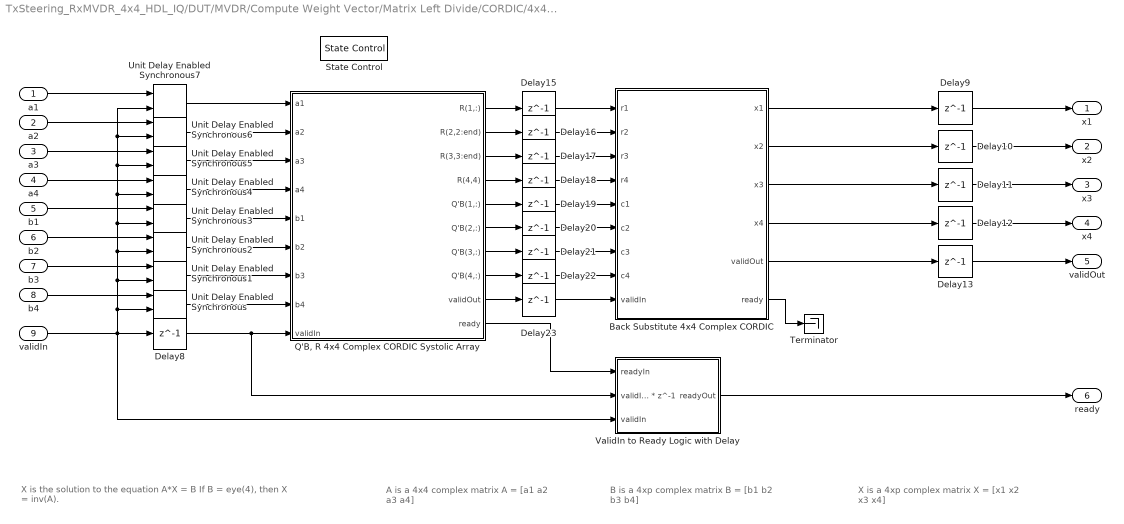
== system TxSteering_RxMVDR_4x4_HDL_IQ/DUT/MVDR/Compute Weight Vector/Matrix Left Divide/CORDIC/4x4 Complex CORDIC Matrix Left Divide ==
  note: X is a 4xp complex matrix
      |
      | X = [x1
      | x2
      | x3
      | x4]
  note: B is a 4xp complex matrix
      |
      | B = [b1
      | b2
      | b3
      | b4]
  note: A is a 4x4 complex matrix
      |
      | A = [a1
      | a2
      | a3
      | a4]
  note: X is the solution to the equation A*X = B
      |
      | If B = eye(4), then X = inv(A).
  a1 : Inport
  a2 : Inport  Port=2
  a3 : Inport  Port=3
  a4 : Inport  Port=4
  b1 : Inport  Port=5
  b2 : Inport  Port=6
  b3 : Inport  Port=7
  b4 : Inport  Port=8
  validIn : Inport  Port=9
  Back Substitute 4x4 Complex CORDIC : Subsystem  TreatAsAtomicUnit=on  mask{NumberOfCORDICIterations=NumberOfCORDICIterations, OutputPrototype=OutputPrototype}
      mask prompts: NumberOfCORDICIterations "Number of CORDIC Iterations"; OutputPrototype "Output Prototype"
  Delay{8..13,15..23} (15 alike) : Delay  DelayLength=1
  "Q'B, R 4x4 Complex CORDIC Systolic Array" : Subsystem  TreatAsAtomicUnit=on  mask{NumberOfCORDICIterations=NumberOfCORDICIterations}
      mask prompts: NumberOfCORDICIterations "Number of CORDIC Iterations"
  State Control : StateControl  StateControl=Synchronous
  Terminator : Terminator
  Unit Delay Enabled Synchronous{,1..7} (8 alike) : hdlsllib/Discrete/Unit Delay Enabled Synchronous  InitialCondition=0.0  SampleTime=-1
      settings: SourceProductBaseCode=SL
  ValidIn to Ready Logic with Delay : Subsystem
  x1 : Outport  VectorParamsAs1DForOutWhenUnconnected=off
  x2 : Outport  Port=2  VectorParamsAs1DForOutWhenUnconnected=off
  x3 : Outport  Port=3  VectorParamsAs1DForOutWhenUnconnected=off
  x4 : Outport  Port=4  VectorParamsAs1DForOutWhenUnconnected=off
  validOut : Outport  Port=5  VectorParamsAs1DForOutWhenUnconnected=off
  ready : Outport  Port=6  VectorParamsAs1DForOutWhenUnconnected=off
  wires:
  "Q'B, R 4x4 Complex CORDIC Systolic Array"/10(ready) -> ValidIn to Ready Logic with Delay/1(readyIn)
  Delay23/1 -> Back Substitute 4x4 Complex CORDIC/9(validIn)
  Delay22/1 -> Back Substitute 4x4 Complex CORDIC/8(c4)
  Delay21/1 -> Back Substitute 4x4 Complex CORDIC/7(c3)
  Delay20/1 -> Back Substitute 4x4 Complex CORDIC/6(c2)
  Delay19/1 -> Back Substitute 4x4 Complex CORDIC/5(c1)
  Delay18/1 -> Back Substitute 4x4 Complex CORDIC/4(r4)
  Delay17/1 -> Back Substitute 4x4 Complex CORDIC/3(r3)
  Delay16/1 -> Back Substitute 4x4 Complex CORDIC/2(r2)
  Delay15/1 -> Back Substitute 4x4 Complex CORDIC/1(r1)
  Back Substitute 4x4 Complex CORDIC/6(ready) -> Terminator/1
  Back Substitute 4x4 Complex CORDIC/5(validOut) -> Delay13/1
  ValidIn to Ready Logic with Delay/1(readyOut) -> ready/1
  "Q'B, R 4x4 Complex CORDIC Systolic Array"/9(validOut) -> Delay23/1
  "Q'B, R 4x4 Complex CORDIC Systolic Array"/8(Q'B(4,:)) -> Delay22/1
  "Q'B, R 4x4 Complex CORDIC Systolic Array"/7(Q'B(3,:)) -> Delay21/1
  "Q'B, R 4x4 Complex CORDIC Systolic Array"/6(Q'B(2,:)) -> Delay20/1
  "Q'B, R 4x4 Complex CORDIC Systolic Array"/5(Q'B(1,:)) -> Delay19/1
  "Q'B, R 4x4 Complex CORDIC Systolic Array"/4(R(4,4)) -> Delay18/1
  "Q'B, R 4x4 Complex CORDIC Systolic Array"/3(R(3,3:end)) -> Delay17/1
  "Q'B, R 4x4 Complex CORDIC Systolic Array"/2(R(2,2:end)) -> Delay16/1
  "Q'B, R 4x4 Complex CORDIC Systolic Array"/1(R(1,:)) -> Delay15/1
  Back Substitute 4x4 Complex CORDIC/4(x4) -> Delay12/1
  Back Substitute 4x4 Complex CORDIC/3(x3) -> Delay11/1
  Back Substitute 4x4 Complex CORDIC/1(x1) -> Delay9/1
  Back Substitute 4x4 Complex CORDIC/2(x2) -> Delay10/1
  Delay13/1 -> validOut/1
  Delay12/1 -> x4/1
  Delay11/1 -> x3/1
  Delay10/1 -> x2/1
  Delay9/1 -> x1/1
  Unit Delay Enabled Synchronous7/1 -> "Q'B, R 4x4 Complex CORDIC Systolic Array"/1(a1)
  Unit Delay Enabled Synchronous6/1 -> "Q'B, R 4x4 Complex CORDIC Systolic Array"/2(a2)
  Unit Delay Enabled Synchronous5/1 -> "Q'B, R 4x4 Complex CORDIC Systolic Array"/3(a3)
  Unit Delay Enabled Synchronous4/1 -> "Q'B, R 4x4 Complex CORDIC Systolic Array"/4(a4)
  Unit Delay Enabled Synchronous3/1 -> "Q'B, R 4x4 Complex CORDIC Systolic Array"/5(b1)
  Unit Delay Enabled Synchronous2/1 -> "Q'B, R 4x4 Complex CORDIC Systolic Array"/6(b2)
  Unit Delay Enabled Synchronous1/1 -> "Q'B, R 4x4 Complex CORDIC Systolic Array"/7(b3)
  Unit Delay Enabled Synchronous/1 -> "Q'B, R 4x4 Complex CORDIC Systolic Array"/8(b4)
  Delay8/1 -> "Q'B, R 4x4 Complex CORDIC Systolic Array"/9(validIn), ValidIn to Ready Logic with Delay/2(validIn * z^-1)
  validIn/1 -> Delay8/1, ValidIn to Ready Logic with Delay/3(validIn), Unit Delay Enabled Synchronous7/2, Unit Delay Enabled Synchronous6/2, Unit Delay Enabled Synchronous5/2, Unit Delay Enabled Synchronous4/2, Unit Delay Enabled Synchronous3/2, Unit Delay Enabled Synchronous2/2, Unit Delay Enabled Synchronous1/2, Unit Delay Enabled Synchronous/2
  b4/1 -> Unit Delay Enabled Synchronous/1
  b3/1 -> Unit Delay Enabled Synchronous1/1
  b2/1 -> Unit Delay Enabled Synchronous2/1
  b1/1 -> Unit Delay Enabled Synchronous3/1
  a4/1 -> Unit Delay Enabled Synchronous4/1
  a3/1 -> Unit Delay Enabled Synchronous5/1
  a2/1 -> Unit Delay Enabled Synchronous6/1
  a1/1 -> Unit Delay Enabled Synchronous7/1

== system TxSteering_RxMVDR_4x4_HDL_IQ/DUT/MVDR/Compute Weight Vector/Matrix Left Divide/QR Solver/Emulate CORDIC Ready ==
  In1 : Inport
  Compare To Constant : simulink/Logic and Bit Operations/Compare To Constant  relop===  const=NumberOfCORDICIterations+7  OutDataTypeStr=boolean
  Compare To Zero : simulink/Logic and Bit Operations/Compare To Zero  relop===  OutDataTypeStr=boolean
  Compare To Zero1 : simulink/Logic and Bit Operations/Compare To Zero  relop=>  OutDataTypeStr=boolean
  HDL Counter : hdlsllib/Sources/HDL Counter  CountType=Free running  CountInit=0  CountStep=1  CountMax=25  CountFromType=Initial value  CountFrom=0  CountResetPort=on  CountLoadPort=off  CountEnbPort=on  CountDirPort=off  CountDataType=Unsigned  CountWordLen=32  CountFracLen=0  CountSampTime=1
  Logical Operator : Logic  Operator=OR  AllPortsSameDT=off  OutDataTypeStr=boolean
  Out1 : Outport
  wires:
  HDL Counter/1 -> Compare To Zero1/1, Compare To Constant/1, Compare To Zero/1
  Compare To Constant/1 -> HDL Counter/1
  Compare To Zero1/1 -> Logical Operator/2
  Logical Operator/1 -> HDL Counter/2
  In1/1 -> Logical Operator/1
  Compare To Zero/1 -> Out1/1

== system TxSteering_RxMVDR_4x4_HDL_IQ/DUT/MVDR/Compute Weight Vector/Matrix Left Divide/QR Solver/Subsystem ==
  In1 : Inport
  In2 : Inport  Port=2
  Enable : EnablePort
  QR Solver : dspsolvers/QR Solver  SimulateUsing=Interpreted execution
      settings: SourceProductBaseCode=DS
  Out1 : Outport
  wires:
  In2/1 -> QR Solver/2
  QR Solver/1 -> Out1/1
  In1/1 -> QR Solver/1

== system TxSteering_RxMVDR_4x4_HDL_IQ/DUT/MVDR/Form Covariance Matrix/Matrix Multiply Partitioned/Partition x_conj/Partition x ==
  x : Inport  Partition=on  PartitionDimension=1  PartitionWidth=1  PartitionOffset=0
  x_conj_elem : Inport  Port=2
  For Each : ForEach  DisableCoverage=on
  HDL Complex Multiply : Subsystem  mask(HDL Complex Multiplier (3 Multiply, 5 Add)){D1=2, D2=1, D3=1, D4=1, D5=1}
      mask help:
      | Xilinx devices:
      | - Set D1 = 1 or 2 to trade off speed & FF resources
      | - Set D2-D5 = 1 to fully leverage DSP48 pipelines
      | - Use sync reset
      |
      | Intel FPGAs:
      | - Set D1 = 1 or 2 depending on device family
      | - Set D5 = 1; D2, D3, D4 = 0
      | - Use async reset
      mask init:
      | delay = D1+D2+D3+D4+D5;
      mask Display:
      | fprintf('Delay=%d',delay);
      | port_label('input',1,'z1');
      | port_label('input',2,'z2');
  C_col : Outport  ConcatenationDimension=1
  wires:
  x/1 -> HDL Complex Multiply/1(In1)
  x_conj_elem/1 -> HDL Complex Multiply/2(In2)
  HDL Complex Multiply/1(Out1) -> C_col/1

== system TxSteering_RxMVDR_4x4_HDL_IQ/DUT/MVDR/Normalize Response/MVDR Weight Update/Inner Product/Element-wise complex product ==
  u : Inport  Partition=on  PartitionDimension=1  PartitionWidth=1  PartitionOffset=0
  v : Inport  Port=2  Partition=on  PartitionDimension=1  PartitionWidth=1  PartitionOffset=0
  For Each : ForEach  DisableCoverage=on
  HDL Complex Multiply : Subsystem  mask(HDL Complex Multiplier (3 Multiply, 5 Add)){D1=2, D2=1, D3=1, D4=1, D5=1}
      mask help:
      | Xilinx devices:
      | - Set D1 = 1 or 2 to trade off speed & FF resources
      | - Set D2-D5 = 1 to fully leverage DSP48 pipelines
      | - Use sync reset
      |
      | Intel FPGAs:
      | - Set D1 = 1 or 2 depending on device family
      | - Set D5 = 1; D2, D3, D4 = 0
      | - Use async reset
      mask init:
      | delay = D1+D2+D3+D4+D5;
      mask Display:
      | fprintf('Delay=%d',delay);
      | port_label('input',1,'z1');
      | port_label('input',2,'z2');
  y : Outport  ConcatenationDimension=1
  wires:
  v/1 -> HDL Complex Multiply/2(In2)
  HDL Complex Multiply/1(Out1) -> y/1
  u/1 -> HDL Complex Multiply/1(In1)

== system TxSteering_RxMVDR_4x4_HDL_IQ/DUT/MVDR/Normalize Response/MVDR Weight Update/Inner Product/Tree Sum with Distributed Pipelining ==
  In1 : Inport
  Delay3 : Delay  DelayLength=ceil(log2(numArrayElements))
  Tree Sum of Elements : Sum  Inputs=+  OutDataTypeStr=Inherit: Same as first input  LockScale=on
  Out1 : Outport
  wires:
  Delay3/1 -> Out1/1
  In1/1 -> Tree Sum of Elements/1
  Tree Sum of Elements/1 -> Delay3/1

== system TxSteering_RxMVDR_4x4_HDL_IQ/DUT/MVDR/Subsystem/RepackageInput/Bitconcat/For Each Subsystem ==
  In1 : Inport  Partition=on  PartitionDimension=1  PartitionWidth=1  PartitionOffset=0
  Bit Concat : hdlsllib/Logic and Bit Operations/Bit Concat  numInputs=2
  Complex to Real-Imag : ComplexToRealImag
  For Each : ForEach  DisableCoverage=on
  Out1 : Outport  ConcatenationDimension=1
  wires:
  In1/1 -> Complex to Real-Imag/1
  Complex to Real-Imag/1 -> Bit Concat/2
  Complex to Real-Imag/2 -> Bit Concat/1
  Bit Concat/1 -> Out1/1
